simulink model "Lab_10"  (R2023a)
settings: Solver=VariableStepAuto  StartTime=0.0  StopTime=10.0  RelTol=1e-3
libraries: spsMonostableLib x1, spsSawtoothGeneratorLib x1
settings Model: Creator=mluser  LastModifiedBy=mluser

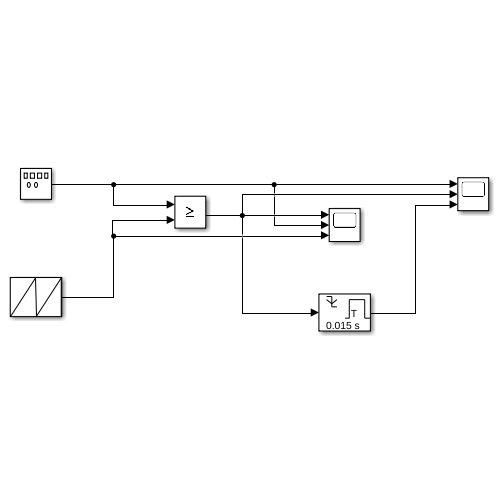
[thumbnail: Simulink's stored preview of the top-level diagram]
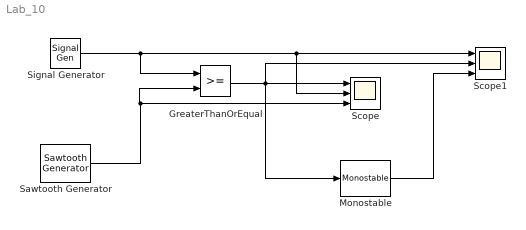
== system Lab_10 ==
  GreaterThanOrEqual : RelationalOperator  OutDataTypeStr=boolean  RndMeth=Simplest  InputSameDT=off
  Monostable : spsMonostableLib/Monostable  EdgeDetect=Falling  PulseDuration=0.015  ic=0  Ts=0
      settings: LibrarySourceBlock=sps_lib/Control/Monostable
  Sawtooth Generator : spsSawtoothGeneratorLib/Sawtooth Generator  Freq=1  Phase=0  Ts=0
  Scope : Scope  NumInputPorts=3
  Scope1 : Scope  NumInputPorts=3
  Signal Generator : SignalGenerator  Frequency=0.5  Units=rad/sec
  wires:
  Signal Generator/1 -> Scope1/1, Scope/2, GreaterThanOrEqual/1
  Sawtooth Generator/1 -> Scope/3, GreaterThanOrEqual/2
  GreaterThanOrEqual/1 -> Scope/1, Monostable/1, Scope1/2
  Monostable/1 -> Scope1/3
